simulink model "CheckValve"  (R2024b)
settings: Solver=VariableStepAuto  StartTime=0.0  StopTime=10.0  RelTol=1e-3
values from neighbouring files (symbols this model uses):
  params = struct    [BranchAndBound.m]    (also in Optimization.m; Parameters.m = struct(); RectangularOptimization.m; RoundingPI.m)
libraries: simulink x1
settings Model: Creator=jackson  LastModifiedBy=jackson

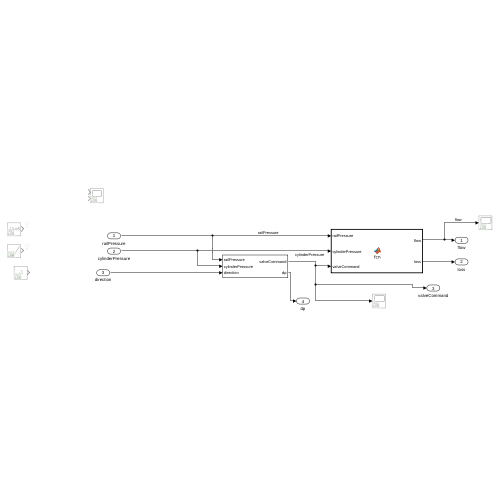
[thumbnail: Simulink's stored preview of the top-level diagram]
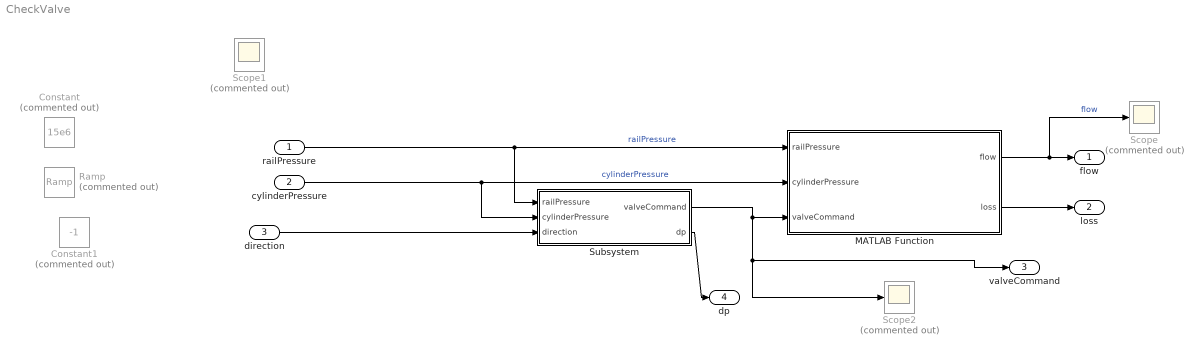
== system CheckValve ==
  railPressure : Inport
  cylinderPressure : Inport  Port=2
  direction : Inport  Port=3
  Constant : Constant  Commented=on  Value=15e6
  Constant1 : Constant  Commented=on  Value=-1
  MATLAB Function : MATLAB Function  TreatAsAtomicUnit=on
  Ramp : simulink/Sources/Ramp  Commented=on  slope=-1e6  start=0  InitialOutput=20e6
  Scope : Scope  Commented=on
  Scope1 : Scope  Commented=on  NumInputPorts=2
  Scope2 : Scope  Commented=on
  Subsystem : Subsystem
  flow : Outport
  loss : Outport  Port=2
  valveCommand : Outport  Port=3
  dp : Outport  Port=4
  wires:
  railPressure/1 -> Subsystem/1(railPressure), MATLAB Function/1(railPressure)  "railPressure"
  cylinderPressure/1 -> MATLAB Function/2(cylinderPressure), Subsystem/2(cylinderPressure)  "cylinderPressure"
  direction/1 -> Subsystem/3(direction)
  MATLAB Function/1(flow) -> Scope/1, flow/1  "flow"
  MATLAB Function/2(loss) -> loss/1
  Subsystem/1(valveCommand) -> valveCommand/1, Scope2/1, MATLAB Function/3(valveCommand)
  Subsystem/2(dp) -> dp/1

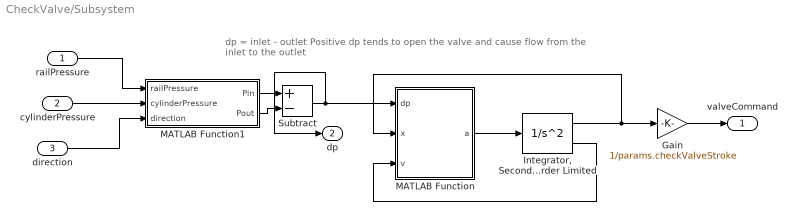
== system CheckValve/Subsystem ==
  note: dp = inlet - outlet
      | Positive dp tends to open the valve and cause flow from the inlet to the outlet
  railPressure : Inport
  cylinderPressure : Inport  Port=2
  direction : Inport  Port=3
  Gain : Gain  Gain=1/params.checkValveStroke
  "Integrator, Second-Order Limited" : SecondOrderIntegrator  LimitX=on  UpperLimitX=params.checkValveStroke  LowerLimitX=0  LimitDXDT=on
  MATLAB Function : MATLAB Function  TreatAsAtomicUnit=on
  MATLAB Function1 : MATLAB Function  TreatAsAtomicUnit=on
  Subtract : Sum  Inputs=+-
  valveCommand : Outport
  dp : Outport  Port=2
  wires:
  "Integrator, Second-Order Limited"/1 -> MATLAB Function/2(x), Gain/1
  "Integrator, Second-Order Limited"/2 -> MATLAB Function/3(v)
  MATLAB Function/1(a) -> "Integrator, Second-Order Limited"/1
  MATLAB Function1/2(Pout) -> Subtract/2
  Subtract/1 -> dp/1, MATLAB Function/1(dp)
  railPressure/1 -> MATLAB Function1/1(railPressure)
  MATLAB Function1/1(Pin) -> Subtract/1
  cylinderPressure/1 -> MATLAB Function1/2(cylinderPressure)
  direction/1 -> MATLAB Function1/3(direction)
  Gain/1 -> valveCommand/1

== matlab function CheckValve/Subsystem/MATLAB Function1 ==
  data: railPressure input; Pin output; cylinderPressure input; direction input; Pout output
function [Pin,Pout] = fcn(railPressure, cylinderPressure, direction)
% positive "direction" allows flow into the cylinder
if direction > 0
    Pin = railPressure;
    Pout = cylinderPressure;
else
    Pin = cylinderPressure;
    Pout = railPressure;
end

== matlab function CheckValve/Subsystem/MATLAB Function ==
  data: dp input; a output; x input; v input; params parameter
function a = fcn(dp,x,v,params)

stroke = params.checkValveStroke;
A = pi*(3*.0254)^2;
m = 7939*A*stroke;
Pc = params.checkValveCrackingPressure;
k = Pc*A/stroke;
c = 2*sqrt(k*m); % critically damped
springPreset = Pc*A ;

a = 1/m * (dp*A -k*x - c*v - springPreset);

== matlab function CheckValve/MATLAB Function ==
  data: railPressure input; flow output; cylinderPressure input; valveCommand input; params parameter; loss output
function [flow,loss] = fcn(railPressure,cylinderPressure,valveCommand,params)
dP = railPressure-cylinderPressure;
flow = valveCommand*params.valveConstant*sqrt(abs(dP))*sign(dP);
loss = (dP)*flow;
